simulink model "controle_estabilidade_lqr2"  (R2021b)
settings: Solver=ode45  StartTime=0.0  StopTime=1000  MaxStep=0.4  RelTol=1e-3
values from neighbouring files (symbols this model uses):
  b = 5.16e-06    [parametros.mat]    (also in parametros2.mat)
  J = [0.00216966666667  0  0; 0  0.00216966666667  0; 0  0  0.00216966666667]    [parametros.mat]    (also in parametros2.mat)
  Jr = 3e-06    [parametros.mat]    (also in parametros2.mat)
  K3_lqr = [-0.00411479129773 -0.978555007624 4.80596451432 -707.681734274]    [parametros2.mat]
  Kiw = 0.0467    [parametros.mat]    (also in parametros2.mat)
  Km = 0.0264    [parametros.mat]    (also in parametros2.mat)
  Kpw = 0.1772    [parametros.mat]    (also in parametros2.mat)
libraries: sharedutil x1, aerolibutil x1
settings Model: Creator=JRRL  LastModifiedBy=JRRL

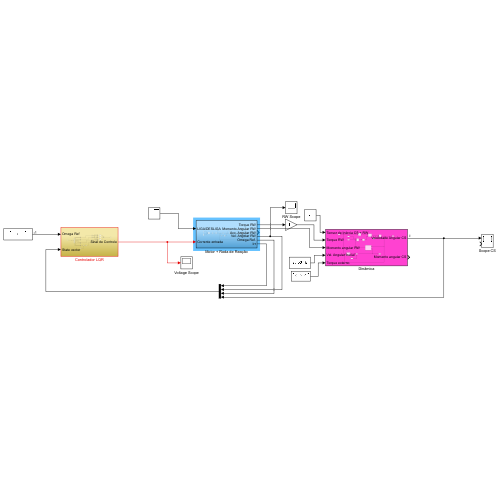
[thumbnail: Simulink's stored preview of the top-level diagram]
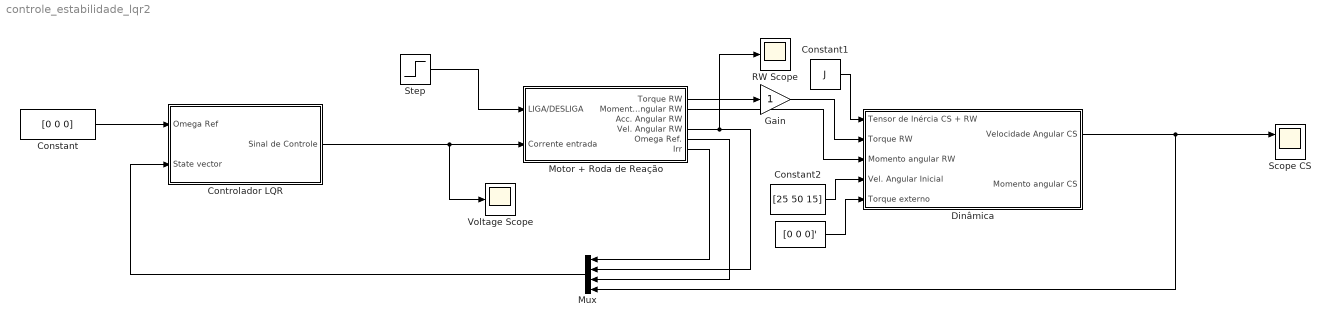
== system controle_estabilidade_lqr2 ==
  " " : Constant  Value=[0 0 0]'
  Constant : Constant  Value=[0 0 0]
  Constant1 : Constant  Value=J
  Constant2 : Constant  Value=[25 50 15]
  Controlador LQR : Subsystem
  Dinâmica : Subsystem
  Gain : Gain
  Motor + Roda de Reação : Subsystem
  Mux : Mux
  RW Scope : Scope
  Scope CS : Scope  NumInputPorts=2
  Step : Step  Time=100  Before=1  SampleTime=0
  Voltage Scope : Scope
  wires:
  Constant1/1 -> Dinâmica/1(Tensor de Inércia CS + RW)
  Dinâmica/1(Velocidade Angular CS) -> Mux/4, Scope CS/1
  Constant2/1 -> Dinâmica/4(Vel. Angular Inicial)
  " "/1 -> Dinâmica/5(Torque externo)
  Mux/1 -> Controlador LQR/2(State vector)
  Constant/1 -> Controlador LQR/1(Omega Ref)
  Controlador LQR/1(Sinal de Controle) -> Motor + Roda de Reação/2(Corrente entrada), Voltage Scope/1
  Motor + Roda de Reação/1(Torque RW) -> Gain/1
  Motor + Roda de Reação/2(Momento Angular RW) -> Dinâmica/3(Momento angular RW)
  Step/1 -> Motor + Roda de Reação/1(LIGA/DESLIGA)
  Motor + Roda de Reação/6(Irr) -> Mux/1
  Motor + Roda de Reação/4(Vel. Angular RW) -> RW Scope/1, Mux/2
  Motor + Roda de Reação/5(Omega Ref.) -> Mux/3
  Gain/1 -> Dinâmica/2(Torque RW)

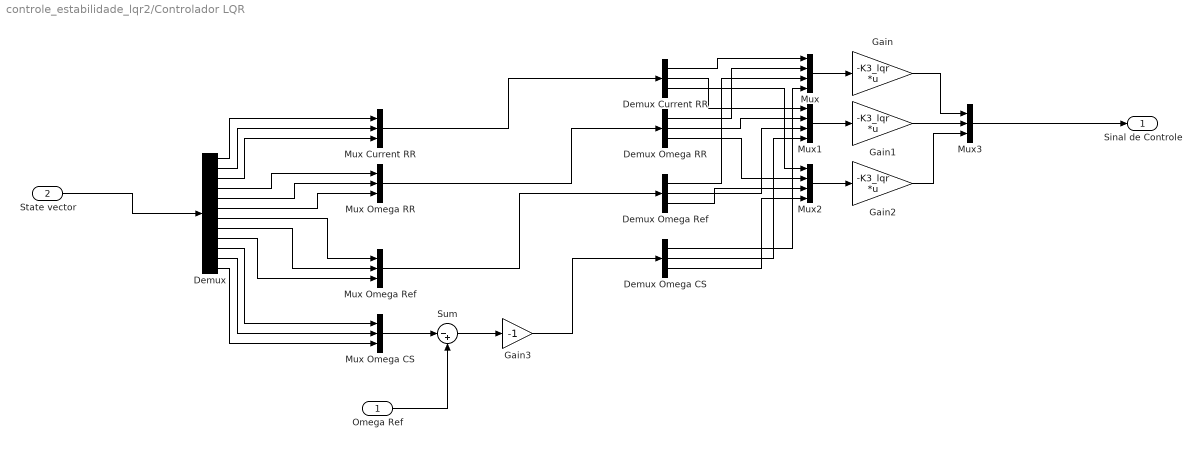
== system controle_estabilidade_lqr2/Controlador LQR ==
  Omega Ref : Inport
  State vector : Inport  Port=2
  Demux : Demux  Outputs=12
  Demux Current RR : Demux  Outputs=3
  Demux Omega CS : Demux  Outputs=3
  Demux Omega RR : Demux  Outputs=3
  Demux Omega Ref : Demux  Outputs=3
  Gain : Gain  Gain=-K3_lqr  Multiplication=Matrix(K*u)
  Gain1 : Gain  Gain=-K3_lqr  Multiplication=Matrix(K*u)
  Gain2 : Gain  Gain=-K3_lqr  Multiplication=Matrix(K*u)
  Gain3 : Gain  Gain=-1
  Mux : Mux
  Mux Current RR : Mux  Inputs=3
  Mux Omega CS : Mux  Inputs=3
  Mux Omega RR : Mux  Inputs=3
  Mux Omega Ref : Mux  Inputs=3
  Mux1 : Mux
  Mux2 : Mux
  Mux3 : Mux  Inputs=3
  Sum : Sum  Inputs=|-+
  Sinal de Controle : Outport
  wires:
  Mux/1 -> Gain/1
  Mux1/1 -> Gain1/1
  Mux2/1 -> Gain2/1
  Gain1/1 -> Mux3/2
  Gain2/1 -> Mux3/3
  Gain/1 -> Mux3/1
  Mux3/1 -> Sinal de Controle/1
  Demux/1 -> Mux Current RR/1
  Demux/2 -> Mux Current RR/2
  Demux/3 -> Mux Current RR/3
  Demux/5 -> Mux Omega RR/2
  Demux/6 -> Mux Omega RR/3
  Demux/4 -> Mux Omega RR/1
  Mux Current RR/1 -> Demux Current RR/1
  Demux Current RR/1 -> Mux/1
  Demux Current RR/2 -> Mux1/1
  Demux Current RR/3 -> Mux2/1
  Demux Omega RR/1 -> Mux/2
  Demux Omega RR/2 -> Mux1/2
  Demux Omega RR/3 -> Mux2/2
  State vector/1 -> Demux/1
  Demux/7 -> Mux Omega Ref/1
  Demux/8 -> Mux Omega Ref/2
  Demux/9 -> Mux Omega Ref/3
  Mux Omega RR/1 -> Demux Omega RR/1
  Mux Omega Ref/1 -> Demux Omega Ref/1
  Demux Omega Ref/1 -> Mux/3
  Demux Omega Ref/2 -> Mux1/3
  Demux Omega Ref/3 -> Mux2/3
  Demux/10 -> Mux Omega CS/1
  Demux/11 -> Mux Omega CS/2
  Demux/12 -> Mux Omega CS/3
  Mux Omega CS/1 -> Sum/1
  Omega Ref/1 -> Sum/2
  Sum/1 -> Gain3/1
  Demux Omega CS/1 -> Mux/4
  Demux Omega CS/2 -> Mux1/4
  Demux Omega CS/3 -> Mux2/4
  Gain3/1 -> Demux Omega CS/1

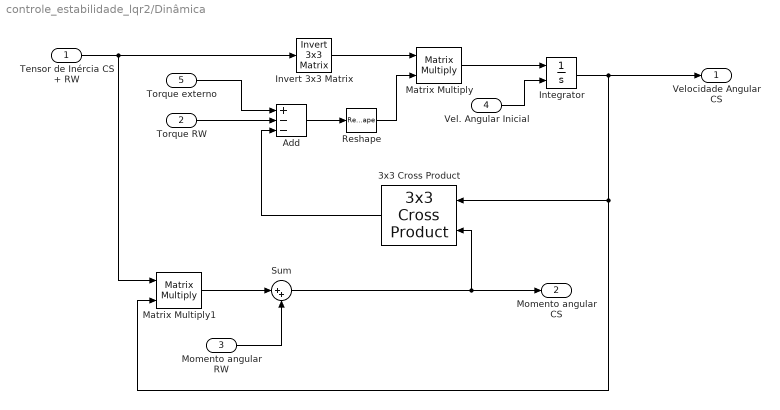
== system controle_estabilidade_lqr2/Dinâmica ==
  Tensor de Inércia CS + RW : Inport
  Torque RW : Inport  Port=2
  Momento angular RW : Inport  Port=3
  Vel. Angular Inicial : Inport  Port=4
  Torque externo : Inport  Port=5
  3x3 Cross Product : sharedutil/3x3 Cross Product  aMode=aMode
      settings: SourceProductBaseCode=AE,PW,DR,MT,UV,VE
  Add : Sum  Inputs=+--
  Integrator : Integrator  InitialConditionSource=external
  Invert 3x3 Matrix : aerolibutil/Invert  3x3 Matrix
  Matrix Multiply : Product  Multiplication=Matrix(*)
  Matrix Multiply1 : Product  Multiplication=Matrix(*)
  Reshape : Reshape  OutputDimensionality=Column vector (2-D)
  Sum : Sum  Inputs=|++
  Velocidade Angular CS : Outport
  Momento angular CS : Outport  Port=2
  wires:
  Sum/1 -> Momento angular CS/1, 3x3 Cross Product/2
  3x3 Cross Product/1 -> Add/3
  Invert 3x3 Matrix/1 -> Matrix Multiply/1
  Integrator/1 -> Velocidade Angular CS/1, Matrix Multiply1/2, 3x3 Cross Product/1
  Matrix Multiply/1 -> Integrator/1
  Momento angular RW/1 -> Sum/2
  Torque RW/1 -> Add/2
  Tensor de Inércia CS + RW/1 -> Matrix Multiply1/1, Invert 3x3 Matrix/1
  Torque externo/1 -> Add/1
  Vel. Angular Inicial/1 -> Integrator/2
  Add/1 -> Reshape/1
  Matrix Multiply1/1 -> Sum/1
  Reshape/1 -> Matrix Multiply/2

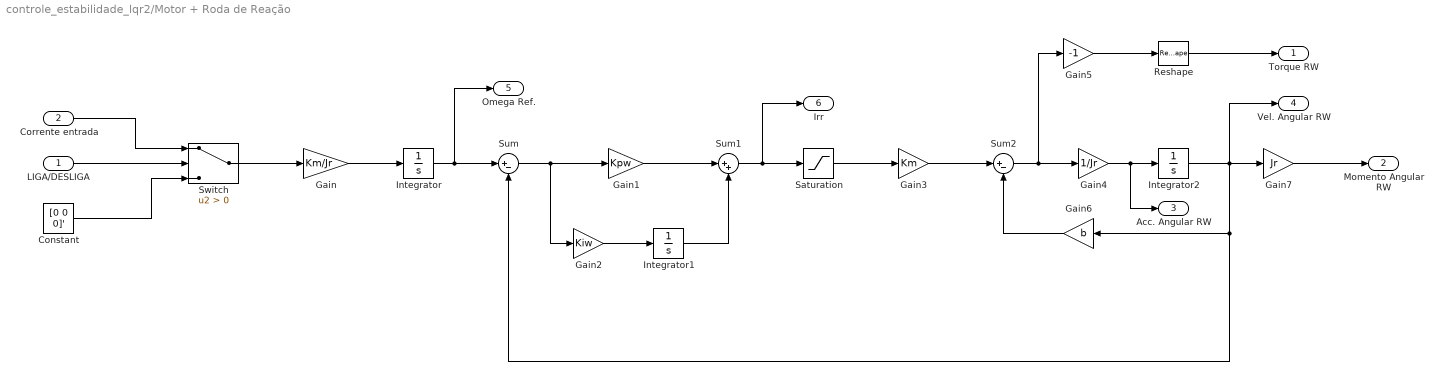
== system controle_estabilidade_lqr2/Motor + Roda de Reação ==
  LIGA/DESLIGA : Inport
  Corrente entrada : Inport  Port=2
  Constant : Constant  Value=[0 0 0]'
  Gain : Gain  Gain=Km/Jr
  Gain1 : Gain  Gain=Kpw
  Gain2 : Gain  Gain=Kiw
  Gain3 : Gain  Gain=Km
  Gain4 : Gain  Gain=1/Jr
  Gain5 : Gain  Gain=-1
  Gain6 : Gain  Gain=b
  Gain7 : Gain  Gain=Jr
  Integrator : Integrator
  Integrator1 : Integrator
  Integrator2 : Integrator
  Reshape : Reshape  OutputDimensionality=Column vector (2-D)
  Saturation : Saturate
  Sum : Sum  Inputs=|+-
  Sum1 : Sum  Inputs=|++
  Sum2 : Sum  Inputs=|+-
  Switch : Switch  Criteria=u2 > Threshold
  Torque RW : Outport
  Momento Angular RW : Outport  Port=2
  Acc. Angular RW : Outport  Port=3
  Vel. Angular RW : Outport  Port=4
  Omega Ref. : Outport  Port=5
  Irr : Outport  Port=6
  wires:
  Saturation/1 -> Gain3/1
  Gain1/1 -> Sum1/1
  Sum/1 -> Gain2/1, Gain1/1
  Reshape/1 -> Torque RW/1
  Sum1/1 -> Irr/1, Saturation/1
  Gain2/1 -> Integrator1/1
  Sum2/1 -> Gain5/1, Gain4/1
  Integrator2/1 -> Vel. Angular RW/1, Sum/2, Gain6/1, Gain7/1
  Gain4/1 -> Acc. Angular RW/1, Integrator2/1
  Gain7/1 -> Momento Angular RW/1
  Gain6/1 -> Sum2/2
  Gain5/1 -> Reshape/1
  Integrator1/1 -> Sum1/2
  Gain3/1 -> Sum2/1
  Integrator/1 -> Omega Ref./1, Sum/1
  Gain/1 -> Integrator/1
  LIGA/DESLIGA/1 -> Switch/2
  Corrente entrada/1 -> Switch/1
  Constant/1 -> Switch/3
  Switch/1 -> Gain/1
